simulink subsystem "Mk2Sensing"  (R2023b)
settings: Solver=VariableStepAuto  StartTime=0.0  StopTime=10.0  RelTol=1e-3
undefined symbols (not defined in the file): Joint1_B, Joint1_F, Joint2_B, Joint2_F, Joint3_B, Joint3_F, MCU_Ts, Phase1_Pos, Phase2_Pos, Phase3_Pos, Phase_Neg
libraries: nesl_utility x12, fl_lib x12, sm_lib x3
settings Model: DataDictionary=neck_mk3.sldd  EnableAccessToBaseWorkspace=off  Creator=upattacini  LastModifiedBy=upattacini

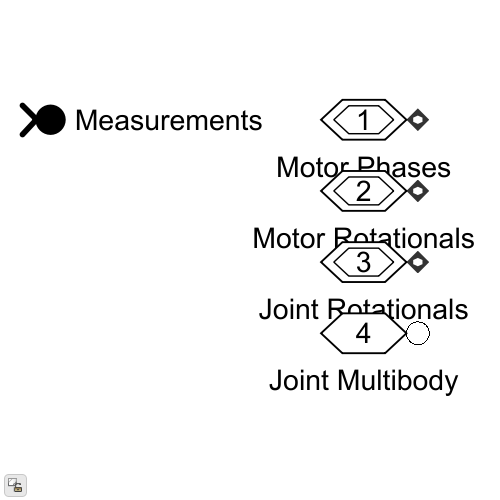
[thumbnail: Simulink's stored preview of the top-level diagram]
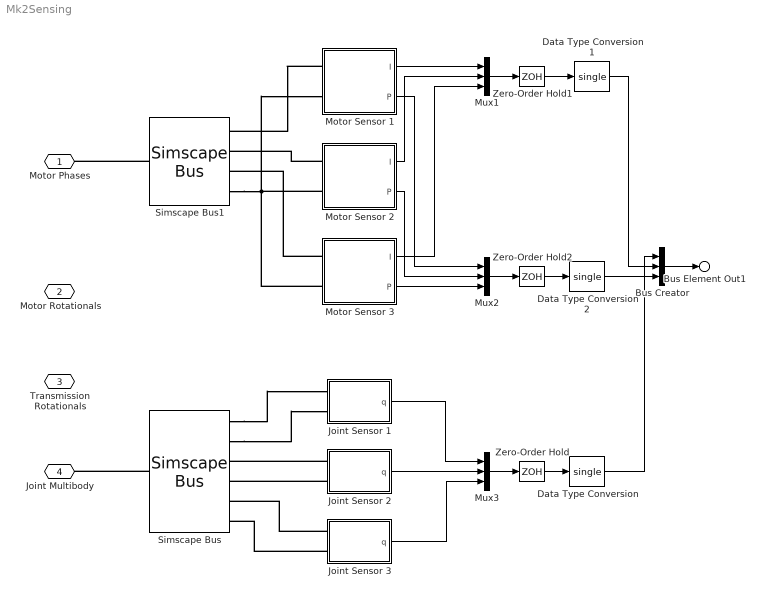
== system Mk2Sensing ==
  Bus Creator : BusCreator  Inputs=3  OutDataTypeStr=Bus: Data_Measurements  NonVirtualBus=on
      settings: InheritFromInputs=off
  Data Type Conversion : DataTypeConversion  OutDataTypeStr=single  SaturateOnIntegerOverflow=off  RndMeth=Floor
  Data Type Conversion1 : DataTypeConversion  OutDataTypeStr=single  SaturateOnIntegerOverflow=off  RndMeth=Floor
  Data Type Conversion2 : DataTypeConversion  OutDataTypeStr=single  SaturateOnIntegerOverflow=off  RndMeth=Floor
  Joint Sensor 1 : Subsystem
  Joint Sensor 2 : Subsystem
  Joint Sensor 3 : Subsystem
  Motor Sensor 1 : Subsystem
  Motor Sensor 2 : Subsystem
  Motor Sensor 3 : Subsystem
  Mux1 : Mux  Inputs=3
  Mux2 : Mux  Inputs=3
  Mux3 : Mux  Inputs=3
  Simscape Bus : SimscapeBus  HierarchyStrings=Joint1_B;Joint1_F;Joint2_B;Joint2_F;Joint3_B;Joint3_F  ConnectionType=Bus: Physical_JointMultibody
  Simscape Bus1 : SimscapeBus  HierarchyStrings=Phase1_Pos;Phase2_Pos;Phase3_Pos;Phase_Neg  ConnectionType=Bus: Physical_MotorPhases
  Zero-Order Hold : ZeroOrderHold  SampleTime=MCU_Ts
  Zero-Order Hold1 : ZeroOrderHold  SampleTime=MCU_Ts
  Zero-Order Hold2 : ZeroOrderHold  SampleTime=MCU_Ts
  Motor Phases : PMIOPort  Side=Right  ConnectionType=Bus: Physical_MotorPhases
  Motor Rotationals : PMIOPort  Port=2  Side=Right  ConnectionType=Bus: Physical_MotorRotationals
  Transmission Rotationals : PMIOPort  Port=3  Side=Right  ConnectionType=Bus: Physical_TransmissionRotationals
  Joint Multibody : PMIOPort  Port=4  Side=Right
  Bus Element Out1 : Outport  PortName=Measurements
  wires:
  Zero-Order Hold/1 -> Data Type Conversion/1
  Bus Creator/1 -> Bus Element Out1/1
  Mux3/1 -> Zero-Order Hold/1
  Data Type Conversion/1 -> Bus Creator/1
  Motor Sensor 1/1(I) -> Mux1/1
  Motor Sensor 2/1(I) -> Mux1/2
  Motor Sensor 3/1(I) -> Mux1/3
  Motor Sensor 3/2(P) -> Mux2/3
  Motor Sensor 2/2(P) -> Mux2/2
  Motor Sensor 1/2(P) -> Mux2/1
  Mux1/1 -> Zero-Order Hold1/1
  Mux2/1 -> Zero-Order Hold2/1
  Zero-Order Hold1/1 -> Data Type Conversion1/1
  Zero-Order Hold2/1 -> Data Type Conversion2/1
  Data Type Conversion1/1 -> Bus Creator/2
  Data Type Conversion2/1 -> Bus Creator/3
  Joint Sensor 1/1(q) -> Mux3/1
  Joint Sensor 2/1(q) -> Mux3/2
  Joint Sensor 3/1(q) -> Mux3/3
  connections:
  Motor Sensor 2/LConn2 -- Motor Sensor 3/LConn2 -- Simscape Bus1/LConn4 -- Motor Sensor 1/LConn2
  Simscape Bus/RConn1 -- Joint Multibody/RConn1
  Simscape Bus1/RConn1 -- Motor Phases/RConn1
  Motor Sensor 1/LConn1 -- Simscape Bus1/LConn1
  Motor Sensor 2/LConn1 -- Simscape Bus1/LConn2
  Motor Sensor 3/LConn1 -- Simscape Bus1/LConn3
  Simscape Bus/LConn1 -- Joint Sensor 1/LConn1
  Simscape Bus/LConn2 -- Joint Sensor 1/LConn2
  Joint Sensor 2/LConn1 -- Simscape Bus/LConn3
  Joint Sensor 2/LConn2 -- Simscape Bus/LConn4
  Joint Sensor 3/LConn1 -- Simscape Bus/LConn5
  Joint Sensor 3/LConn2 -- Simscape Bus/LConn6

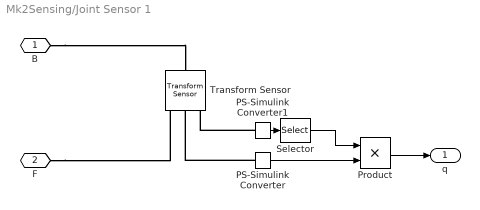
== system Mk2Sensing/Joint Sensor 1 ==
  PS-Simulink Converter : nesl_utility/PS-Simulink Converter  PhysicalDomain=network_engine_domain  SubClassName=ps_output  LeftPortType=input  RightPortType=output  PseudoPeriodic=off  Frequencies=[]  VectorFormat=inherit  Unit=deg  AffineConversion=off
  PS-Simulink Converter1 : nesl_utility/PS-Simulink Converter  PhysicalDomain=network_engine_domain  SubClassName=ps_output  LeftPortType=input  RightPortType=output  PseudoPeriodic=off  Frequencies=[]  VectorFormat=1-D array  Unit=1  AffineConversion=off
  Product : Product
  Selector : Selector  InputPortWidth=3  IndexOptions=Index vector (dialog)  Indices=3  OutputSizes=1
  Transform Sensor : sm_lib/Frames and Transforms/Transform Sensor  MeasurementFrame=Base  RotationSequence=XYX  SenseAngle=on  SenseAxis=on  SenseQ=off  SenseR=off  SenseRotationSequence=off  SenseOmegaX=off  SenseOmegaY=off  SenseOmegaZ=off  SenseOmega=off  SenseQDot=off  SenseRDot=off  SenseRotationSequenceDot=off  SenseAlphaX=off  SenseAlphaY=off  SenseAlphaZ=off  SenseAlpha=off  SenseQDDot=off  SenseRDDot=off  SenseX=off  SenseY=off  SenseZ=off  SenseXYZ=off  SenseRad=off  SenseAzim=off  SenseDist=off  SenseInc=off  SenseXDot=off  SenseYDot=off  SenseZDot=off  SenseXYZDot=off  SenseRadDot=off  SenseAzimDot=off  SenseDistDot=off  SenseIncDot=off  SenseXDDot=off  SenseYDDot=off  SenseZDDot=off  SenseXYZDDot=off  SenseRadDDot=off  SenseAzimDDot=off  SenseDistDDot=off  SenseIncDDot=off
  B : PMIOPort  Side=Left
  F : PMIOPort  Port=2  Side=Left
  q : Outport
  wires:
  Product/1 -> q/1
  Selector/1 -> Product/1
  PS-Simulink Converter/1 -> Product/2
  PS-Simulink Converter1/1 -> Selector/1
  connections:
  PS-Simulink Converter1/LConn1 -- Transform Sensor/RConn3
  B/RConn1 -- Transform Sensor/LConn1
  PS-Simulink Converter/LConn1 -- Transform Sensor/RConn2
  F/RConn1 -- Transform Sensor/RConn1

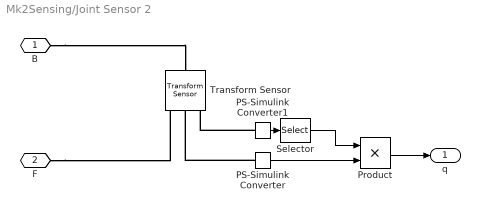
== system Mk2Sensing/Joint Sensor 2 ==
  PS-Simulink Converter : nesl_utility/PS-Simulink Converter  PhysicalDomain=network_engine_domain  SubClassName=ps_output  LeftPortType=input  RightPortType=output  PseudoPeriodic=off  Frequencies=[]  VectorFormat=inherit  Unit=deg  AffineConversion=off
  PS-Simulink Converter1 : nesl_utility/PS-Simulink Converter  PhysicalDomain=network_engine_domain  SubClassName=ps_output  LeftPortType=input  RightPortType=output  PseudoPeriodic=off  Frequencies=[]  VectorFormat=1-D array  Unit=1  AffineConversion=off
  Product : Product
  Selector : Selector  InputPortWidth=3  IndexOptions=Index vector (dialog)  Indices=3  OutputSizes=1
  Transform Sensor : sm_lib/Frames and Transforms/Transform Sensor  MeasurementFrame=Base  RotationSequence=XYX  SenseAngle=on  SenseAxis=on  SenseQ=off  SenseR=off  SenseRotationSequence=off  SenseOmegaX=off  SenseOmegaY=off  SenseOmegaZ=off  SenseOmega=off  SenseQDot=off  SenseRDot=off  SenseRotationSequenceDot=off  SenseAlphaX=off  SenseAlphaY=off  SenseAlphaZ=off  SenseAlpha=off  SenseQDDot=off  SenseRDDot=off  SenseX=off  SenseY=off  SenseZ=off  SenseXYZ=off  SenseRad=off  SenseAzim=off  SenseDist=off  SenseInc=off  SenseXDot=off  SenseYDot=off  SenseZDot=off  SenseXYZDot=off  SenseRadDot=off  SenseAzimDot=off  SenseDistDot=off  SenseIncDot=off  SenseXDDot=off  SenseYDDot=off  SenseZDDot=off  SenseXYZDDot=off  SenseRadDDot=off  SenseAzimDDot=off  SenseDistDDot=off  SenseIncDDot=off
  B : PMIOPort  Side=Left
  F : PMIOPort  Port=2  Side=Left
  q : Outport
  wires:
  PS-Simulink Converter1/1 -> Selector/1
  PS-Simulink Converter/1 -> Product/2
  Selector/1 -> Product/1
  Product/1 -> q/1
  connections:
  F/RConn1 -- Transform Sensor/RConn1
  PS-Simulink Converter/LConn1 -- Transform Sensor/RConn2
  B/RConn1 -- Transform Sensor/LConn1
  PS-Simulink Converter1/LConn1 -- Transform Sensor/RConn3

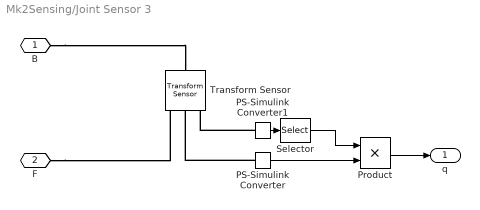
== system Mk2Sensing/Joint Sensor 3 ==
  PS-Simulink Converter : nesl_utility/PS-Simulink Converter  PhysicalDomain=network_engine_domain  SubClassName=ps_output  LeftPortType=input  RightPortType=output  PseudoPeriodic=off  Frequencies=[]  VectorFormat=inherit  Unit=deg  AffineConversion=off
  PS-Simulink Converter1 : nesl_utility/PS-Simulink Converter  PhysicalDomain=network_engine_domain  SubClassName=ps_output  LeftPortType=input  RightPortType=output  PseudoPeriodic=off  Frequencies=[]  VectorFormat=1-D array  Unit=1  AffineConversion=off
  Product : Product
  Selector : Selector  InputPortWidth=3  IndexOptions=Index vector (dialog)  Indices=3  OutputSizes=1
  Transform Sensor : sm_lib/Frames and Transforms/Transform Sensor  MeasurementFrame=Base  RotationSequence=XYX  SenseAngle=on  SenseAxis=on  SenseQ=off  SenseR=off  SenseRotationSequence=off  SenseOmegaX=off  SenseOmegaY=off  SenseOmegaZ=off  SenseOmega=off  SenseQDot=off  SenseRDot=off  SenseRotationSequenceDot=off  SenseAlphaX=off  SenseAlphaY=off  SenseAlphaZ=off  SenseAlpha=off  SenseQDDot=off  SenseRDDot=off  SenseX=off  SenseY=off  SenseZ=off  SenseXYZ=off  SenseRad=off  SenseAzim=off  SenseDist=off  SenseInc=off  SenseXDot=off  SenseYDot=off  SenseZDot=off  SenseXYZDot=off  SenseRadDot=off  SenseAzimDot=off  SenseDistDot=off  SenseIncDot=off  SenseXDDot=off  SenseYDDot=off  SenseZDDot=off  SenseXYZDDot=off  SenseRadDDot=off  SenseAzimDDot=off  SenseDistDDot=off  SenseIncDDot=off
  B : PMIOPort  Side=Left
  F : PMIOPort  Port=2  Side=Left
  q : Outport
  wires:
  Product/1 -> q/1
  Selector/1 -> Product/1
  PS-Simulink Converter/1 -> Product/2
  PS-Simulink Converter1/1 -> Selector/1
  connections:
  PS-Simulink Converter1/LConn1 -- Transform Sensor/RConn3
  B/RConn1 -- Transform Sensor/LConn1
  PS-Simulink Converter/LConn1 -- Transform Sensor/RConn2
  F/RConn1 -- Transform Sensor/RConn1

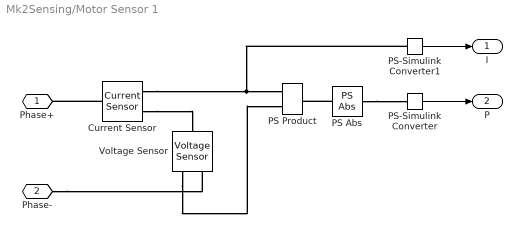
== system Mk2Sensing/Motor Sensor 1 ==
  Current Sensor : fl_lib/Electrical/Electrical Sensors/Current Sensor
  PS Abs : fl_lib/Physical Signals/Nonlinear Operators/PS Abs
      settings: InternalSimscapePortConfiguration="{\"Bottom\":[],\"Left\":[{\"id\":\"I\",\"label\":\"\",\"type\":\"input\"}],\"Right\":[{\"id\":\"O\",\"label\":\"\",\"type\":\"output\"}],\"Top\":[]}"
  PS Product : fl_lib/Physical Signals/Functions/PS Product
  PS-Simulink Converter : nesl_utility/PS-Simulink Converter  PhysicalDomain=network_engine_domain  SubClassName=ps_output  LeftPortType=input  RightPortType=output  PseudoPeriodic=off  Frequencies=[]  VectorFormat=inherit  Unit=inherit  AffineConversion=off
  PS-Simulink Converter1 : nesl_utility/PS-Simulink Converter  PhysicalDomain=network_engine_domain  SubClassName=ps_output  LeftPortType=input  RightPortType=output  PseudoPeriodic=off  Frequencies=[]  VectorFormat=inherit  Unit=inherit  AffineConversion=off
  Voltage Sensor : fl_lib/Electrical/Electrical Sensors/Voltage Sensor
  Phase+ : PMIOPort  Side=Left
  Phase- : PMIOPort  Port=2  Side=Left
  I : Outport
  P : Outport  Port=2
  wires:
  PS-Simulink Converter/1 -> P/1
  PS-Simulink Converter1/1 -> I/1
  connections:
  PS Abs/RConn1 -- PS-Simulink Converter/LConn1
  PS Abs/LConn1 -- PS Product/RConn1
  Phase-/RConn1 -- Voltage Sensor/RConn2
  PS-Simulink Converter1/LConn1 -- Current Sensor/RConn1 -- PS Product/LConn1
  Current Sensor/LConn1 -- Phase+/RConn1
  Voltage Sensor/RConn1 -- PS Product/LConn2
  Current Sensor/RConn2 -- Voltage Sensor/LConn1

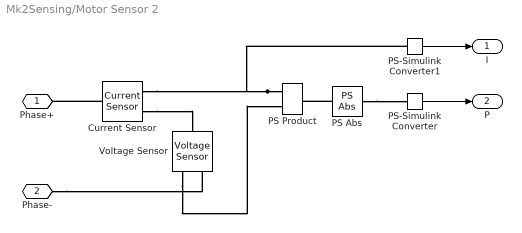
== system Mk2Sensing/Motor Sensor 2 ==
  Current Sensor : fl_lib/Electrical/Electrical Sensors/Current Sensor
  PS Abs : fl_lib/Physical Signals/Nonlinear Operators/PS Abs
      settings: InternalSimscapePortConfiguration="{\"Bottom\":[],\"Left\":[{\"id\":\"I\",\"label\":\"\",\"type\":\"input\"}],\"Right\":[{\"id\":\"O\",\"label\":\"\",\"type\":\"output\"}],\"Top\":[]}"
  PS Product : fl_lib/Physical Signals/Functions/PS Product
  PS-Simulink Converter : nesl_utility/PS-Simulink Converter  PhysicalDomain=network_engine_domain  SubClassName=ps_output  LeftPortType=input  RightPortType=output  PseudoPeriodic=off  Frequencies=[]  VectorFormat=inherit  Unit=inherit  AffineConversion=off
  PS-Simulink Converter1 : nesl_utility/PS-Simulink Converter  PhysicalDomain=network_engine_domain  SubClassName=ps_output  LeftPortType=input  RightPortType=output  PseudoPeriodic=off  Frequencies=[]  VectorFormat=inherit  Unit=inherit  AffineConversion=off
  Voltage Sensor : fl_lib/Electrical/Electrical Sensors/Voltage Sensor
  Phase+ : PMIOPort  Side=Left
  Phase- : PMIOPort  Port=2  Side=Left
  I : Outport
  P : Outport  Port=2
  wires:
  PS-Simulink Converter1/1 -> I/1
  PS-Simulink Converter/1 -> P/1
  connections:
  Current Sensor/RConn2 -- Voltage Sensor/LConn1
  Voltage Sensor/RConn1 -- PS Product/LConn2
  Current Sensor/LConn1 -- Phase+/RConn1
  PS Product/LConn1 -- Current Sensor/RConn1 -- PS-Simulink Converter1/LConn1
  Phase-/RConn1 -- Voltage Sensor/RConn2
  PS Abs/LConn1 -- PS Product/RConn1
  PS Abs/RConn1 -- PS-Simulink Converter/LConn1

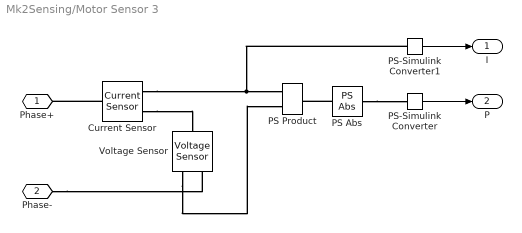
== system Mk2Sensing/Motor Sensor 3 ==
  Current Sensor : fl_lib/Electrical/Electrical Sensors/Current Sensor
  PS Abs : fl_lib/Physical Signals/Nonlinear Operators/PS Abs
      settings: InternalSimscapePortConfiguration="{\"Bottom\":[],\"Left\":[{\"id\":\"I\",\"label\":\"\",\"type\":\"input\"}],\"Right\":[{\"id\":\"O\",\"label\":\"\",\"type\":\"output\"}],\"Top\":[]}"
  PS Product : fl_lib/Physical Signals/Functions/PS Product
  PS-Simulink Converter : nesl_utility/PS-Simulink Converter  PhysicalDomain=network_engine_domain  SubClassName=ps_output  LeftPortType=input  RightPortType=output  PseudoPeriodic=off  Frequencies=[]  VectorFormat=inherit  Unit=inherit  AffineConversion=off
  PS-Simulink Converter1 : nesl_utility/PS-Simulink Converter  PhysicalDomain=network_engine_domain  SubClassName=ps_output  LeftPortType=input  RightPortType=output  PseudoPeriodic=off  Frequencies=[]  VectorFormat=inherit  Unit=inherit  AffineConversion=off
  Voltage Sensor : fl_lib/Electrical/Electrical Sensors/Voltage Sensor
  Phase+ : PMIOPort  Side=Left
  Phase- : PMIOPort  Port=2  Side=Left
  I : Outport
  P : Outport  Port=2
  wires:
  PS-Simulink Converter/1 -> P/1
  PS-Simulink Converter1/1 -> I/1
  connections:
  PS Abs/RConn1 -- PS-Simulink Converter/LConn1
  PS Abs/LConn1 -- PS Product/RConn1
  Phase-/RConn1 -- Voltage Sensor/RConn2
  PS-Simulink Converter1/LConn1 -- Current Sensor/RConn1 -- PS Product/LConn1
  Current Sensor/LConn1 -- Phase+/RConn1
  Voltage Sensor/RConn1 -- PS Product/LConn2
  Current Sensor/RConn2 -- Voltage Sensor/LConn1
